simulink model "stateflow_test"  (R2025b)
settings: Solver=VariableStepAuto  StartTime=0.0  StopTime=10.0  RelTol=1e-3
libraries: simulink x2
settings Model: Creator=David  LastModifiedBy=David

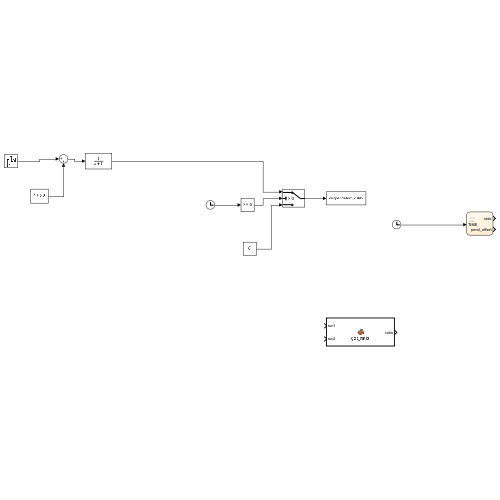
[thumbnail: Simulink's stored preview of the top-level diagram]
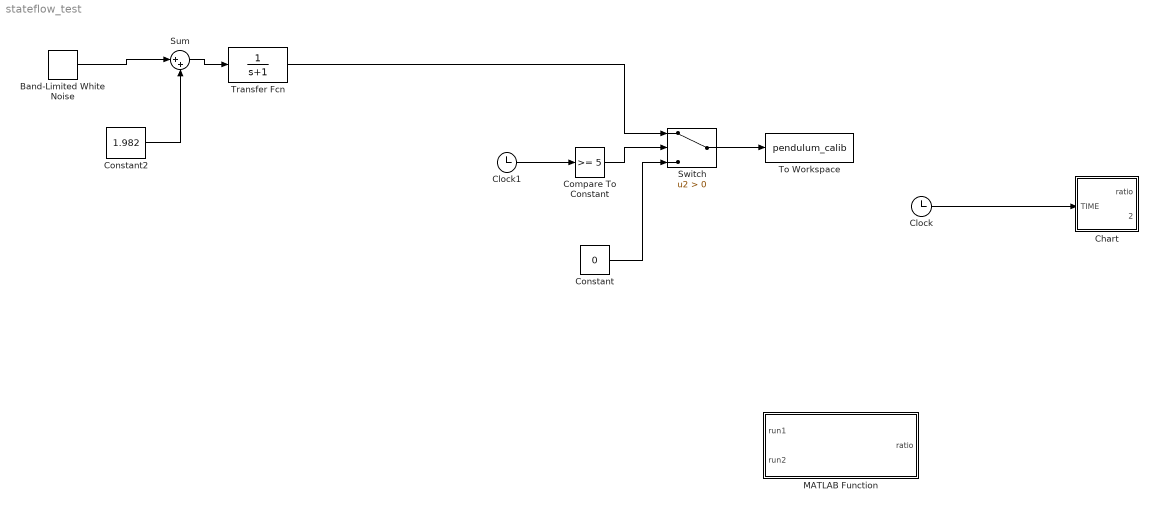
== system stateflow_test ==
  Band-Limited White Noise : simulink/Sources/Band-Limited White Noise  Cov=[0.1]  Ts=0.1  seed=[23341]
  Chart : Stateflow chart  TreatAsAtomicUnit=on
  Clock : Clock
  Clock1 : Clock
  Compare To Constant : simulink/Logic and Bit Operations/Compare To Constant  relop=>=  const=5  OutDataTypeStr=boolean
  Constant : Constant  Value=0
  Constant2 : Constant  Value=1.982
  MATLAB Function : MATLAB Function  TreatAsAtomicUnit=on
  Sum : Sum  Inputs=|++
  Switch : Switch  Criteria=u2 > Threshold  SaturateOnIntegerOverflow=off  InputSameDT=off
  To Workspace : ToWorkspace  VariableName=pendulum_calib  SaveFormat=Timeseries  SampleTime=-1
  Transfer Fcn : TransferFcn  Denominator=[1 1]
  wires:
  Clock/1 -> Chart/1(TIME)
  Clock1/1 -> Compare To Constant/1
  Compare To Constant/1 -> Switch/2
  Constant/1 -> Switch/3
  Constant2/1 -> Sum/2
  Band-Limited White Noise/1 -> Sum/1
  Transfer Fcn/1 -> Switch/1
  Sum/1 -> Transfer Fcn/1
  Switch/1 -> To Workspace/1

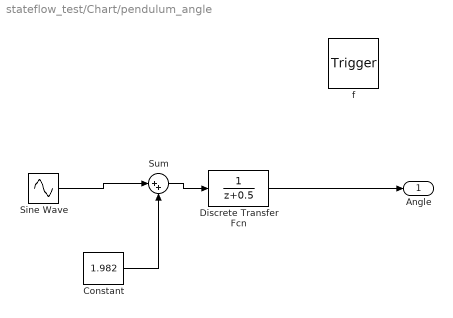
== system stateflow_test/Chart/pendulum_angle ==
  f : TriggerPort  TriggerType=function-call  VariantControl=(inherit)
      settings: CopyFcn=Stateflow.SLINSF.SimulinkMan.removeBlockPreDeleteFcn  PreDeleteFcn=Stateflow.SLINSF.SimulinkMan.unsafePredeleteFcn
  Constant : Constant  Value=1.982
  Discrete Transfer Fcn : DiscreteTransferFcn
  Sine Wave : Sin
  Sum : Sum  Inputs=|++
  Angle : Outport
  wires:
  Discrete Transfer Fcn/1 -> Angle/1
  Constant/1 -> Sum/2
  Sum/1 -> Discrete Transfer Fcn/1
  Sine Wave/1 -> Sum/1

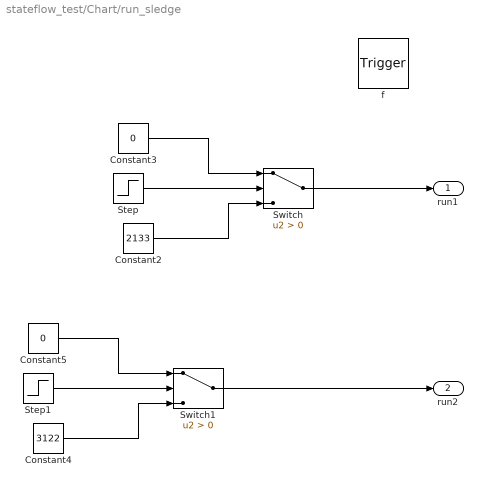
== system stateflow_test/Chart/run_sledge ==
  f : TriggerPort  TriggerType=function-call  VariantControl=(inherit)
      settings: CopyFcn=Stateflow.SLINSF.SimulinkMan.removeBlockPreDeleteFcn  PreDeleteFcn=Stateflow.SLINSF.SimulinkMan.unsafePredeleteFcn
  Constant2 : Constant  Value=2133
  Constant3 : Constant  Value=0
  Constant4 : Constant  Value=3122
  Constant5 : Constant  Value=0
  Step : Step  Time=4  Before=1  After=0
  Step1 : Step  Time=4  Before=1  After=0
  Switch : Switch  Criteria=u2 > Threshold  SaturateOnIntegerOverflow=off  InputSameDT=off
  Switch1 : Switch  Criteria=u2 > Threshold  SaturateOnIntegerOverflow=off  InputSameDT=off
  run1 : Outport
  run2 : Outport  Port=2
  wires:
  Switch/1 -> run1/1
  Switch1/1 -> run2/1
  Step/1 -> Switch/2
  Constant2/1 -> Switch/3
  Constant3/1 -> Switch/1
  Constant5/1 -> Switch1/1
  Step1/1 -> Switch1/2
  Constant4/1 -> Switch1/3

== matlab function stateflow_test/MATLAB Function ==
  data: run1 input; ratio output; run2 input
function ratio = get_ratio(run1, run2)

distance = 0.114;
avg_counts = (run1+run2)/2;

ratio = distance / avg_counts;

end

== stateflow chart stateflow_test/Chart ==
  state Calibration
    state Pendulum
      entry:
      pend_offset = pendulum_angle()
    state Sledge
      during:
      [run1, run2] = run_sledge()
      exit:
      ratio = get_ratio(run1, run2)
      STEP = 3
    state Center
      exit:
      STEP = 4
    (default) -> Pendulum : {pend_offset = 0;}
    Pendulum -> Sledge : [TIME>4]
        | {ratio = 0}
    Sledge -> Center : [STEP == 3]
  state Angle = pendulum_angle [function]
  state [run1, run2]= run_sledge [function]
  data: Angle function_output; run1 function_output; run2 function_output; run1 function_input; run2 function_input; ratio function_output; TIME input; ratio output; pend_offset output; STEP local; run1 local; run2 local
  function ratio = get_ratio(run1, run2):
    | function ratio = get_ratio(run1, run2)
    | 
    | distance = 0.114;
    | avg_counts = (run1+run2)/2;
    | 
    | ratio = distance / avg_counts;
    | 
    | end
